simulink model "problem3"  (R2020b)
settings: Solver=VariableStepAuto  StartTime=0.0  StopTime=tstop  RelTol=1e-3
values from neighbouring files (symbols this model uses):
  a1 = 0.5792    [variables.m]
  b1 = 0.1584    [variables.m]
settings Model: Creator=shweta  LastModifiedBy=shweta
settings DataIOCC: ExternalInput=[t,noise]  LoadExternalInput=on

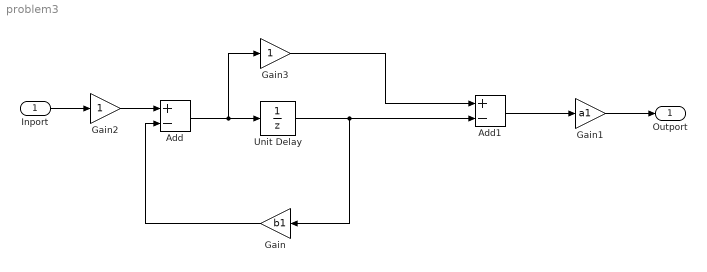
== system problem3 ==
  Inport : Inport
  Add : Sum  Inputs=+-
  Add1 : Sum  Inputs=+-
  Gain : Gain  Gain=b1
  Gain1 : Gain  Gain=a1
  Gain2 : Gain
  Gain3 : Gain
  Unit Delay : UnitDelay  SampleTime=-1  HasFrameUpgradeWarning=on
  Outport : Outport
  wires:
  Unit Delay/1 -> Add1/2, Gain/1
  Gain/1 -> Add/2
  Inport/1 -> Gain2/1
  Gain2/1 -> Add/1
  Add/1 -> Gain3/1, Unit Delay/1
  Add1/1 -> Gain1/1
  Gain1/1 -> Outport/1
  Gain3/1 -> Add1/1
